simulink library "tqd"  (R2021b)
settings: Solver=VariableStepAuto  StartTime=0.0  StopTime=10.0  RelTol=1e-3
undefined symbols (not defined in the file): ATQD_AfterTqMinGain_X_Deg, ATQD_APSCreepBaseTqD_X_kph, ATQD_APSCreepBaseTqD_Y_Deg, ATQD_APSCreepBaseTqR_X_kph, ATQD_APSCreepBaseTqR_Y_Deg, ATQD_APSCreepIterm_X_kph, ATQD_APSCreepIterm_Y_kph, ATQD_APSCreepPterm_X_kph, ATQD_APSCreepPterm_Y_kph, ATQD_APSDecReq_X_kph, ATQD_APSDecReq_Y_mps2, ATQD_APSDecReqCMD_X_kph, ATQD_APSDecReqTs_X_pct, ATQD_APSDecTimeGain_X_Deg, ATQD_APSDecTimeGain_Y_s, ATQD_APSReqLowSpd_X_Deg, ATQD_AutoHoldReleaseBPS_X_Deg, ATQD_AWDLoadTrqnsGain_X_kg, ATQD_AWDLoadTrqnsGain_Y_pct, ATQD_BOSEnBPSPosn_X_kph, ATQD_BOSMap_X_rpm, ATQD_BOSMap_Y_pct, ATQD_CreepBaseTqD_X_kph, ATQD_CreepBaseTqD_Y_Deg, ATQD_CreepBaseTqR_X_kph, ATQD_CreepBaseTqR_Y_Deg, ATQD_CreepBPSDisPosn_X_Deg, ATQD_CreepBPSDisPosnR_X_Deg, ATQD_CreepBPSEnPosn_X_Deg, ATQD_CreepBPSEnPosnR_X_Deg, ATQD_CreepDeltaTq_X_kph, ATQD_CreepIterm_X_kph, ATQD_CreepIterm_Y_kph, ATQD_CreepItermMaxLimit_X_pct, ATQD_CreepPreloadTime_X_kph, ATQD_CreepPreloadTq_X_kph, ATQD_CreepPreloadTq_Y_s, ATQD_CreepProtTq_X_Deg, ATQD_CreepPterm_X_kph, ATQD_CreepPterm_Y_kph, ATQD_CreepRrTqSpRat_X_rpm, ATQD_CreepRrTqSpRat_Y_Nm, ATQD_CreepTargetSpdD_X_pct, ATQD_CreepTargetSpdR_X_pct, ATQD_ECOTqMapD_X_rpm, ATQD_ECOTqMapD_Y_pct, ATQD_EMTqMapD_X_rpm, ATQD_EMTqMapD_Y_pct, ATQD_EOPDTqMapDCon_X_rpm, ATQD_EOPDTqMapDCon_Y_Deg, ATQD_EscapeModePedTq_X_pct, ATQD_EscapeModePedTq_Y_rpm, ATQD_EscapeModePedTqFr_X_pct, ATQD_EscapeModePedTqFr_Y_rpm, ATQD_EstInitVehWeight_X_c, ATQD_FAfterTqCMDGain_X_rpm, ATQD_FAfterTqCMDGain_Y_pct, ATQD_FrLossMAPLowV_X_rpm, ATQD_FrLossMAPLowV_Y_Nm, ATQD_FrMotActReduce_X_rpm ... (+772)
libraries: simulink x211, hcu_lib x179, tqr x3
(part 16 of 28)

== system tqd/TQD/TorqueDemand/TorqueModule/OPD Hold/Deceleration Calculation ==
  VTQD_VehActSpd_kph : Inport
  VVMC_LongAcc_Gps : Inport  Port=2
  VTQD_APSReqTimer_s : Inport  Port=3
  VVMC_EstSlope_Deg : Inport  Port=4
  VTQD_APSDecReqA_flg : Inport  Port=5
  VTQD_AutiHoldRelease_flg : Inport  Port=6
  task_time_s : Inport  Port=7
  VTQD_ActAPSPosn_pct : Inport  Port=8
  AND1 : Logic  Inputs=3  AllPortsSameDT=off  OutDataTypeStr=boolean
  AND4 : Logic  Inputs=3  AllPortsSameDT=off  OutDataTypeStr=boolean
  Add : Sum  Inputs=+-
  Constant1 : Constant  Value=KTQD_APSDecReqMaxTime_s
  Constant13 : Constant  Value=ZERO_FLOAT
  Constant19 : Constant  Value=KTQD_OPDHoldBrkSW_flg
  Constant2 : Constant  Value=KTQD_OPDHoldBrkSW_flg
  Constant21 : Constant  Value=KTQD_OPDHoldDevUpLim_mps2
  Constant22 : Constant  Value=KTQD_OPDHoldDevLowLim_mps2
  Constant43 : Constant  Value=KTQD_APSDecReqMaxSW_flg
  Constant8 : Constant  Value=KVMC_GravityValue_mps2
  Delay : Delay  DelayLength=1
  FirstOrderFilter1 : tqr/TQR/Determine Torque Request/TorqueArbitrament/TorqueSmooth/FirstOrderFilter
  MTQD_APSDecReg_Z_mps2 : Lookup_n-D  BreakpointsForDimension1=ATQD_APSDecReq_Y_mps2  BreakpointsForDimension2=ATQD_APSDecReq_X_kph  Table=MTQD_APSDecReq_Z_mps2  InternalRulePriority=Speed  RndMeth=Simplest  InputSameDT=on
      settings: InputPortMap=u0,u1
  MTQD_APSDecReqCMD_Y_mps2 : Lookup_n-D  NumberOfTableDimensions=1  BreakpointsForDimension1=ATQD_APSDecReqCMD_X_kph  Table=MTQD_APSDecReqCMD_Y_mps2  InternalRulePriority=Speed  RndMeth=Simplest  InputSameDT=on
  MTQD_APSDecReqTs_Y_c : Lookup_n-D  NumberOfTableDimensions=1  BreakpointsForDimension1=ATQD_APSDecReqTs_X_pct  Table=MTQD_APSDecReqTs_Y_c  InternalRulePriority=Speed  RndMeth=Simplest  InputSameDT=on
  MTQD_APSDecTimeGain_Z_c : Lookup_n-D  BreakpointsForDimension1=ATQD_APSDecTimeGain_Y_s  BreakpointsForDimension2=ATQD_APSDecTimeGain_X_Deg  Table=MTQD_APSDecTimeGain_Z_c  InternalRulePriority=Speed  RndMeth=Simplest  InputSameDT=on
      settings: InputPortMap=u0,u1
  Max : MinMax  Function=max  Inputs=2
  NOT{1..3,5} (4 alike) : Logic  Operator=NOT  AllPortsSameDT=off  OutDataTypeStr=boolean
  OR : Logic  Operator=OR  AllPortsSameDT=off  OutDataTypeStr=boolean
  Product : Product
  Product1 : Product
  Product2 : Product
  Relational Operator : RelationalOperator  OutDataTypeStr=boolean  RndMeth=Simplest
  SR_Latch : hcu_lib/Basic_Blocks/SR_Latch
  Saturation Dynamic : simulink/Discontinuities/Saturation Dynamic  OutMin=[]  OutMax=[]  OutDataTypeStr=Inherit: Same as second input  OutDataType=fixdt(1, 16)  OutScaling=2^-10  DoSatur=off
  Switch1 : Switch  Criteria=u2 > Threshold
  Switch3 : Switch  Criteria=u2 > Threshold
  Switch9 : Switch  Criteria=u2 > Threshold
  VTQD_APSDecReq_mps2 : Outport
  wires:
  Saturation Dynamic/1 -> MTQD_APSDecReg_Z_mps2/1  "VTQD_ActOPDHoldAccDev_mps2"
  [VVMC_EstSlope_Deg] -> MTQD_APSDecTimeGain_Z_c/2
  [VTQD_APSDecTimeGain_c] -> Product2/2
  Constant21/1 -> Saturation Dynamic/1
  Product/1 -> Max/1
  Max/1 -> Switch9/1
  MTQD_APSDecReg_Z_mps2/1 -> [VTQD_MapAPSDecReg_mps2]  "VTQD_MapAPSDecReq_mps2"
  Constant13/1 -> Switch3/3
  MTQD_APSDecReqCMD_Y_mps2/1 -> [VTQD_APSDecReqCMD_mps2]  "VTQD_APSDecReqCMD_mps2"
  [VVMC_LongAcc_Gps] -> Product1/1
  [VTQD_MapAPSDecReg_mps2] -> Product2/1
  Delay/1 -> Max/2
  Constant19/1 -> NOT5/1
  Add/1 -> Saturation Dynamic/2
  [VTQD_VehActSpd_kph] -> MTQD_APSDecReg_Z_mps2/2
  [VTQD_APSReqTimer_s] -> MTQD_APSDecTimeGain_Z_c/1
  [VTQD_MapAPSDecReg_mps2] -> Product/1
  Product2/1 -> Switch9/3
  [VTQD_APSDecReq_mps2] -> Delay/1
  Product1/1 -> Add/2
  [VTQD_VehActSpd_kph] -> MTQD_APSDecReqCMD_Y_mps2/1
  MTQD_APSDecTimeGain_Z_c/1 -> [VTQD_APSDecTimeGain_c]  "VTQD_APSDecTimeGain_c"
  [VTQD_APSDecReqA_flg] -> AND4/1
  NOT5/1 -> AND4/2
  [VTQD_APSDecTimeGain_c] -> Product/2
  [VTQD_APSDecReqCMD_mps2] -> Add/1
  Constant22/1 -> Saturation Dynamic/3
  Constant8/1 -> Product1/2
  VTQD_VehActSpd_kph/1 -> [VTQD_VehActSpd_kph]
  VVMC_LongAcc_Gps/1 -> [VVMC_LongAcc_Gps]
  VTQD_APSReqTimer_s/1 -> [VTQD_APSReqTimer_s]
  VVMC_EstSlope_Deg/1 -> [VVMC_EstSlope_Deg]
  VTQD_APSDecReqA_flg/1 -> [VTQD_APSDecReqA_flg]
  [VTQD_APSDecReq_mps2] -> VTQD_APSDecReq_mps2/1
  Constant43/1 -> OR/1
  Relational Operator/1 -> SR_Latch/1
  Constant1/1 -> Relational Operator/2
  [VTQD_APSReqTimer_s] -> Relational Operator/1
  Switch9/1 -> Switch3/1
  [VTQD_AutiHoldRelease_flg] -> SR_Latch/2
  VTQD_AutiHoldRelease_flg/1 -> [VTQD_AutiHoldRelease_flg]
  OR/1 -> Switch9/2  "VTQD_APSDecReqMax_flg"
  SR_Latch/1 -> OR/2
  AND4/1 -> Switch3/2
  NOT2/1 -> AND4/3
  [VTQD_AutiHoldRelease_flg] -> NOT2/1
  NOT1/1 -> AND1/3
  NOT3/1 -> AND1/2
  AND1/1 -> Switch1/2
  Switch3/1 -> Switch1/1, FirstOrderFilter1/1
  Switch1/1 -> [VTQD_APSDecReq_mps2]  "VTQD_APSDecReq_mps2"
  [VTQD_APSDecReqA_flg] -> AND1/1
  Constant2/1 -> NOT3/1
  [VTQD_AutiHoldRelease_flg] -> NOT1/1
  FirstOrderFilter1/1 -> Switch1/3
  [task_time_s] -> FirstOrderFilter1/2
  task_time_s/1 -> [task_time_s]
  VTQD_ActAPSPosn_pct/1 -> [VTQD_ActAPSPosn_pct]
  MTQD_APSDecReqTs_Y_c/1 -> [VTQD_APSDecReqTs_c]  "VTQD_APSDecReqTs_c"
  [VTQD_ActAPSPosn_pct] -> MTQD_APSDecReqTs_Y_c/1
  [VTQD_APSDecReqTs_c] -> FirstOrderFilter1/3

== system tqd/TQD/TorqueDemand/TorqueModule/OPD Hold/OPDHold Request  ==
  VTQD_VehActSpd_kph : Inport
  VTQD_APSStaSys_enum : Inport  Port=2
  VTQD_AutiHoldRelease_flg : Inport  Port=3
  task_time_s : Inport  Port=4
  VVMC_EstSlope_Deg : Inport  Port=5
  AND : Logic  AllPortsSameDT=off  OutDataTypeStr=boolean
  AND1 : Logic  Inputs=3  AllPortsSameDT=off  OutDataTypeStr=boolean
  AND2 : Logic  Operator=OR  AllPortsSameDT=off  OutDataTypeStr=boolean
  AND3 : Logic  AllPortsSameDT=off  OutDataTypeStr=boolean
  Constant1 : Constant  Value=KTQD_APSReqUpSpd_kph
  Constant10 : Constant  Value=KTQD_APSReqDownSpd_kph
  Constant11 : Constant  Value=KTQD_OPDHoldLampDelayTime_s
  Constant12 : Constant  Value=KTQD_OPDHoldLampEnSpd_kph  OutDataTypeStr=single
  Constant13 : Constant  Value=KTQD_OPDHoldLampDisSpd_kph  OutDataTypeStr=single
  Constant2 : Constant  Value=2  OutDataTypeStr=uint8
  Constant3 : Constant  Value=2  OutDataTypeStr=uint8
  Constant4 : Constant  OutDataTypeStr=uint8
  Constant5 : Constant  Value=2  OutDataTypeStr=uint8
  Constant6 : Constant  Value=0  OutDataTypeStr=uint8
  Constant7 : Constant  OutDataTypeStr=uint8
  Constant8 : Constant  OutDataTypeStr=uint8
  Constant9 : Constant  Value=KTQD_APSReqDelayTime_s
  Equal1 : RelationalOperator  Operator=<  OutDataTypeStr=boolean  RndMeth=Simplest
  Equal2 : RelationalOperator  Operator=~=  OutDataTypeStr=boolean  RndMeth=Simplest
  Equal3 : RelationalOperator  Operator===  OutDataTypeStr=boolean  RndMeth=Simplest
  Equal4 : RelationalOperator  Operator===  OutDataTypeStr=boolean  RndMeth=Simplest
  Equal5 : RelationalOperator  Operator===  OutDataTypeStr=boolean  RndMeth=Simplest
  Equal6 : RelationalOperator  Operator=>  OutDataTypeStr=boolean  RndMeth=Simplest
  MTQD_APSReqLowSpd_Y_kph : Lookup_n-D  NumberOfTableDimensions=1  BreakpointsForDimension1=ATQD_APSReqLowSpd_X_Deg  Table=MTQD_APSReqLowSpd_Y_kph  InternalRulePriority=Speed  RndMeth=Simplest  InputSameDT=on
  NOT1 : Logic  Operator=NOT  AllPortsSameDT=off  OutDataTypeStr=boolean
  NOT2 : Logic  Operator=NOT  AllPortsSameDT=off  OutDataTypeStr=boolean
  Relational Operator1 : RelationalOperator  Operator=<  OutDataTypeStr=boolean  RndMeth=Simplest
  Relational Operator2 : RelationalOperator  OutDataTypeStr=boolean  RndMeth=Simplest
  Relational Operator3 : RelationalOperator  Operator=<  OutDataTypeStr=boolean  RndMeth=Simplest
  Relational Operator4 : RelationalOperator  Operator=>  OutDataTypeStr=boolean  RndMeth=Simplest
  Relay : Relay  OnSwitchValue=KTQD_OPDHoldGradeUp_Deg  OffSwitchValue=KTQD_OPDHoldGradeDown_Deg  OutDataTypeStr=boolean
  SR_Latch : hcu_lib/Basic_Blocks/SR_Latch
  SR_Latch1 : hcu_lib/Basic_Blocks/SR_Latch
  Switch : Switch  Criteria=u2 > Threshold
  Switch1 : Switch  Criteria=u2 > Threshold
  Switch2 : Switch  Criteria=u2 > Threshold
  Timer : hcu_lib/Basic_Blocks/Timer
  VTQD_APSReqTimer_s : Outport
  VTQD_APSReq_enum : Outport  Port=2
  VTQD_APSDecReqA_flg : Outport  Port=3
  VTQD_OPDHoldLamp_flg : Outport  Port=4
  wires:
  [task_time_s] -> Timer/3
  Constant4/1 -> Switch1/1
  NOT2/1 -> Timer/2
  Switch2/1 -> [VTQD_APSReq_enum]  "VTQD_APSReq_enum"
  AND/1 -> Switch1/2  "VTQD_APSStasysUp_flg"
  Constant9/1 -> Relational Operator2/2, Timer/4
  Equal3/1 -> AND/2
  Constant6/1 -> Switch1/3
  Timer/1 -> [VTQD_APSReqTimer_s], Relational Operator2/1  "VTQD_APSReqTimer_s"
  Relational Operator2/1 -> Switch2/2
  Constant8/1 -> Switch2/1
  Equal4/1 -> AND1/2
  [VTQD_APSStaSys_enum] -> Equal3/1
  [VTQD_VehActSpd_kph] -> Equal1/1
  Equal5/1 -> [VTQD_APSDecReqA_flg]  "VTQD_APSDecReqA_flg"
  [VTQD_APSReqUpSpd_kph] -> Equal1/2
  NOT1/1 -> AND1/3
  Constant7/1 -> Equal5/2
  [VTQD_APSReq_enum] -> Equal5/1
  Constant2/1 -> Equal3/2
  Switch1/1 -> Switch2/3
  Equal1/1 -> AND/1
  [VTQD_APSStaSys_enum] -> Equal4/1
  [VTQD_VehActSpd_kph] -> Relational Operator1/1
  AND1/1 -> NOT2/1, Timer/1  "VTQD_APSStasysLow_flg"
  Constant5/1 -> Equal4/2
  VTQD_VehActSpd_kph/1 -> [VTQD_VehActSpd_kph]
  VTQD_APSStaSys_enum/1 -> [VTQD_APSStaSys_enum]
  VTQD_AutiHoldRelease_flg/1 -> [VTQD_AutiHoldRelease_flg]
  task_time_s/1 -> [task_time_s]
  [VTQD_APSReqTimer_s] -> VTQD_APSReqTimer_s/1
  [VTQD_APSReq_enum] -> VTQD_APSReq_enum/1
  [VTQD_APSDecReqA_flg] -> VTQD_APSDecReqA_flg/1
  [VTQD_AutiHoldRelease_flg] -> NOT1/1
  VVMC_EstSlope_Deg/1 -> [VVMC_EstSlope_Deg]
  MTQD_APSReqLowSpd_Y_kph/1 -> Relational Operator1/2  "VTQD_APSReqLowSpd_kph"
  [VVMC_EstSlope_Deg] -> MTQD_APSReqLowSpd_Y_kph/1
  SR_Latch/1 -> AND1/1
  Relational Operator1/1 -> SR_Latch/1
  AND2/1 -> SR_Latch/2
  [VTQD_AutiHoldRelease_flg] -> AND2/1
  Constant3/1 -> Equal2/2
  [VTQD_APSStaSys_enum] -> Equal2/1
  Equal2/1 -> AND2/2
  [VVMC_EstSlope_Deg] -> Relay/1
  Relay/1 -> Switch/2  "VTQD_OPDHoldUpDown_flg"
  Constant1/1 -> Switch/1
  Constant10/1 -> Switch/3
  Switch/1 -> [VTQD_APSReqUpSpd_kph]  "VTQD_APSReqUpSpd_kph"
  Constant11/1 -> Equal6/2
  [VTQD_APSReqTimer_s] -> Equal6/1
  [VTQD_OPDHoldLamp_flg] -> VTQD_OPDHoldLamp_flg/1
  [VTQD_VehActSpd_kph] -> Relational Operator3/1
  Relational Operator3/1 -> SR_Latch1/1
  Constant12/1 -> Relational Operator3/2
  [VTQD_VehActSpd_kph] -> Relational Operator4/1
  Constant13/1 -> Relational Operator4/2
  Relational Operator4/1 -> SR_Latch1/2
  Equal6/1 -> AND3/1
  SR_Latch1/1 -> AND3/2  "VTQD_OPDHoldSpdEnLamp_flg"
  AND3/1 -> [VTQD_OPDHoldLamp_flg]  "VTQD_OPDHoldLamp_flg"

== system tqd/TQD/TorqueDemand/TorqueModule/OPD Hold/Parking Requeest Backup ==
  VTQD_APSReq_enum : Inport
  VTQD_APSReqTimer_s : Inport  Port=2
  VTQD_ParkRequest_flg : Inport  Port=3
  task_time_s : Inport  Port=4
  VTQD_AutiHoldRelease_flg : Inport  Port=5
  AND : Logic  AllPortsSameDT=off  OutDataTypeStr=boolean
  AND1 : Logic  AllPortsSameDT=off  OutDataTypeStr=boolean
  AND3 : Logic  Inputs=3  AllPortsSameDT=off  OutDataTypeStr=boolean
  Constant1 : Constant  Value=KTQD_APSReqDelayTime_s
  Constant16 : Constant  OutDataTypeStr=uint8
  Constant17 : Constant  Value=TRUE  OutDataTypeStr=uint8
  Constant2 : Constant  Value=KTQD_APSReqDelayTime_s
  Constant3 : Constant  Value=KTQD_OPDHoldBrkSW_flg
  Constant4 : Constant  Value=KTQD_OPDHoldAllowPark_flg
  Constant5 : Constant  Value=KTQD_OPDHoldAllowPark_s
  Constant6 : Constant  Value=KTQD_OPDHoldAllowGearPSW_flg
  DelayEnable : hcu_lib/Basic_Blocks/DelayEnable
  Equal6 : RelationalOperator  Operator===  OutDataTypeStr=boolean  RndMeth=Simplest
  NOT : Logic  Operator=NOT  AllPortsSameDT=off  OutDataTypeStr=boolean
  OR : Logic  Operator=OR  AllPortsSameDT=off  OutDataTypeStr=boolean
  Relational Operator1 : RelationalOperator  OutDataTypeStr=boolean  RndMeth=Simplest
  Relational Operator6 : RelationalOperator  OutDataTypeStr=boolean  RndMeth=Simplest
  SR_Latch : hcu_lib/Basic_Blocks/SR_Latch
  Switch4 : Switch  Criteria=u2 > Threshold
  VTQD_ActParkRequest_flg : Outport
  VTQD_OPDHoldAllowPark_flg : Outport  Port=2
  wires:
  Constant3/1 -> AND3/2
  Constant1/1 -> Relational Operator6/2
  Equal6/1 -> AND3/1
  [VTQD_APSReq_enum] -> Equal6/1
  Relational Operator6/1 -> AND3/3
  [VTQD_ParkRequest_flg] -> Switch4/3
  Constant17/1 -> Switch4/1
  Constant16/1 -> Equal6/2
  Switch4/1 -> [VTQD_ActParkRequest_flg]  "VTQD_ActParkRequest_flg"
  [VTQD_APSReqTimer_s] -> Relational Operator6/1
  VTQD_APSReq_enum/1 -> [VTQD_APSReq_enum]
  VTQD_APSReqTimer_s/1 -> [VTQD_APSReqTimer_s]
  VTQD_ParkRequest_flg/1 -> [VTQD_ParkRequest_flg]
  [VTQD_ActParkRequest_flg] -> VTQD_ActParkRequest_flg/1
  Constant2/1 -> Relational Operator1/2
  [VTQD_APSReqTimer_s] -> Relational Operator1/1
  task_time_s/1 -> [task_time_s]
  AND/1 -> DelayEnable/1
  Relational Operator1/1 -> AND/1
  Constant4/1 -> AND/2
  Constant5/1 -> DelayEnable/2
  DelayEnable/1 -> SR_Latch/1
  [VTQD_AutiHoldRelease_flg] -> SR_Latch/2
  VTQD_AutiHoldRelease_flg/1 -> [VTQD_AutiHoldRelease_flg]
  SR_Latch/1 -> [VTQD_OPDHoldAllowPark_flg]  "VTQD_OPDHoldAllowPark_flg"
  OR/1 -> Switch4/2
  AND3/1 -> OR/1
  [task_time_s] -> DelayEnable/3
  [VTQD_OPDHoldAllowPark_flg] -> AND1/1
  AND1/1 -> OR/2
  NOT/1 -> AND1/2
  Constant6/1 -> NOT/1
  [VTQD_OPDHoldAllowPark_flg] -> VTQD_OPDHoldAllowPark_flg/1

== system tqd/TQD/TorqueDemand/TorqueModule/OPD Hold/Release Condition ==
  VVMC_EstSlope_Deg : Inport
  VTQD_VehActSpd_kph : Inport  Port=2
  VTQR_NoABSFEDUWhlTqReq_Nm : Inport  Port=3
  VTQR_NoABSREDUWhlTqReq_Nm : Inport  Port=4
  VTQD_ActBPSPosn_pct : Inport  Port=5
  task_time_s : Inport  Port=6
  VTQD_APSReqTimer_s : Inport  Port=7
  VTQD_LowIdleAccPedal_flg : Inport  Port=8
  VTQD_OPDHoldRgnOn2Off_flg : Inport  Port=9
  AND : Logic  Inputs=3  AllPortsSameDT=off  OutDataTypeStr=boolean
  AND1 : Logic  AllPortsSameDT=off  OutDataTypeStr=boolean
  AND2 : Logic  AllPortsSameDT=off  OutDataTypeStr=boolean
  AND3 : Logic  AllPortsSameDT=off  OutDataTypeStr=boolean
  Add : Sum
  Add1 : Sum  Inputs=+-+
  Add6 : Sum
  Add7 : Sum
  Constant1 : Constant  Value=KTQD_APSRelDisTqDev_Nm
  Constant{5,10,23,30} (4 alike) : Constant  Value=ZERO_FLOAT
  Constant2 : Constant  Value=KTQD_OPDHoldDownEnTime_s
  Constant36 : Constant  Value=KTQD_OPDHoldRelDetSpd_kph
  Constant4 : Constant  Value=KTQD_OPDHoldRelTqGain_Nm
  Constant6 : Constant  Value=KTQD_OPDHoldDetRevSpd_kph
  Constant7 : Constant  Value=KTQD_OPDHoldLiftRevSpd_kph
  Constant8 : Constant  Value=KTQD_APSDecReqMaxTime_s
  Constant9 : Constant  Value=KTQD_OPDHoldRelTqGain_Nm
  Delay{,1..3} (4 alike) : Delay  DelayLength=1
  DelayEnable : hcu_lib/Basic_Blocks/DelayEnable
  DelayEnable1 : hcu_lib/Basic_Blocks/DelayEnable
  Detect Increase : simulink/Logic and Bit Operations/Detect Increase  vinit=0.0  OutDataTypeStr=boolean
  Detect Increase1 : simulink/Logic and Bit Operations/Detect Increase  vinit=0.0  OutDataTypeStr=boolean
  Detect Increase2 : simulink/Logic and Bit Operations/Detect Increase  vinit=0.0  OutDataTypeStr=boolean
  MTQD_AutoHoldReleaseBPS_Y_pct : Lookup_n-D  NumberOfTableDimensions=1  BreakpointsForDimension1=ATQD_AutoHoldReleaseBPS_X_Deg  Table=MTQD_AutoHoldReleaseBPS_Y_pct  InternalRulePriority=Speed  RndMeth=Simplest  InputSameDT=on
  MTQD_OPDHoldDownRelDelay_Y_s : Lookup_n-D  NumberOfTableDimensions=1  BreakpointsForDimension1=ATQD_OPDHoldDownRelDelay_X_Deg  Table=MTQD_OPDHoldDownRelDelay_Y_s  InternalRulePriority=Speed  RndMeth=Simplest  InputSameDT=on
  MTQD_OPDHoldRelDetTime_Y_s : Lookup_n-D  NumberOfTableDimensions=1  BreakpointsForDimension1=ATQD_OPDHoldRelDetTime_X_Deg  Table=MTQD_OPDHoldRelDetTime_Y_s  InternalRulePriority=Speed  RndMeth=Simplest  InputSameDT=on
  MTQD_OPDHoldReleaseTq_Y_Nm{,1..3} (4 alike) : Lookup_n-D  NumberOfTableDimensions=1  BreakpointsForDimension1=ATQD_OPDHoldReleaseTq_X_Deg  Table=MTQD_OPDHoldReleaseTq_Y_Nm  InternalRulePriority=Speed  RndMeth=Simplest  InputSameDT=on
  Max : MinMax  Function=max  Inputs=2
  Max1 : MinMax  Function=max  Inputs=2
  Max2 : MinMax  Function=max  Inputs=2
  NOT{,1..5} (6 alike) : Logic  Operator=NOT  AllPortsSameDT=off  OutDataTypeStr=boolean
  OR : Logic  Operator=OR  AllPortsSameDT=off  OutDataTypeStr=boolean
  OR1 : Logic  Operator=OR  AllPortsSameDT=off  OutDataTypeStr=boolean
  OR2 : Logic  Operator=OR  AllPortsSameDT=off  OutDataTypeStr=boolean
  OR3 : Logic  Operator=OR  Inputs=3  AllPortsSameDT=off  OutDataTypeStr=boolean
  Relational Operator : RelationalOperator  Operator=>  OutDataTypeStr=boolean  RndMeth=Simplest
  Relational Operator1 : RelationalOperator  Operator=<=  OutDataTypeStr=boolean  RndMeth=Simplest
  Relational Operator3 : RelationalOperator  Operator=<=  OutDataTypeStr=boolean  RndMeth=Simplest
  Relational Operator4 : RelationalOperator  OutDataTypeStr=boolean  RndMeth=Simplest
  Relational Operator5 : RelationalOperator  Operator=<  OutDataTypeStr=boolean  RndMeth=Simplest
  Relational Operator6 : RelationalOperator  Operator=>  OutDataTypeStr=boolean  RndMeth=Simplest
  Relational Operator7 : RelationalOperator  OutDataTypeStr=boolean  RndMeth=Simplest
  Relational Operator9 : RelationalOperator  OutDataTypeStr=boolean  RndMeth=Simplest
  Relay : Relay  OnSwitchValue=KTQD_OPDHoldGradeUp_Deg  OffSwitchValue=KTQD_OPDHoldGradeDown_Deg  OutDataTypeStr=boolean
  Relay1 : Relay  OnSwitchValue=KTQD_OPDHoldGradeUp_Deg  OffSwitchValue=KTQD_OPDHoldGradeDown_Deg  OutDataTypeStr=boolean
  SR_Latch : hcu_lib/Basic_Blocks/SR_Latch
  SR_Latch1 : hcu_lib/Basic_Blocks/SR_Latch
  Switch{,1..6} (7 alike) : Switch  Criteria=u2 > Threshold
  VTQD_AutoHoldRelease_flg : Outport
  VTQD_OPDHoldEnRel_flg : Outport  Port=2
  VTQD_OPDHoldActRelTq_Nm : Outport  Port=3
  wires:
  VVMC_EstSlope_Deg/1 -> [VVMC_EstSlope_Deg]
  VTQD_VehActSpd_kph/1 -> [VTQD_VehActSpd_kph]
  VTQR_NoABSFEDUWhlTqReq_Nm/1 -> [VTQR_NoABSFEDUWhlTqReq_Nm]
  VTQR_NoABSREDUWhlTqReq_Nm/1 -> [VTQR_NoABSREDUWhlTqReq_Nm]
  VTQD_ActBPSPosn_pct/1 -> [VTQD_ActBPSPosn_pct]
  task_time_s/1 -> [task_time_s]
  [VTQD_AutoHoldRelease_flg] -> VTQD_AutoHoldRelease_flg/1
  [VTQD_OPDHoldEnRel_flg] -> VTQD_OPDHoldEnRel_flg/1
  VTQD_APSReqTimer_s/1 -> [VTQD_APSReqTimer_s]
  VTQD_LowIdleAccPedal_flg/1 -> [VTQD_LowIdleAccPedal_flg]
  VTQD_OPDHoldRgnOn2Off_flg/1 -> [VTQD_OPDHoldRgnOn2Off_flg]
  SR_Latch/1 -> DelayEnable/1  "VTQD_OPDHoldEnRelLatch_flg"
  Detect Increase2/1 -> OR2/1
  Detect Increase1/1 -> SR_Latch1/1
  DelayEnable1/1 -> Switch1/1
  SR_Latch1/1 -> [VTQD_OPDHoldRelReverse_flg]  "VTQD_OPDHoldRelReverse_flg"
  MTQD_OPDHoldDownRelDelay_Y_s/1 -> [VTQD_OPDHoldDownRelDelay_s]  "VTQD_OPDHoldDownRelDelay_s"
  Constant4/1 -> Switch2/1
  [VVMC_EstSlope_Deg] -> MTQD_OPDHoldDownRelDelay_Y_s/1
  [task_time_s] -> DelayEnable1/3
  [VTQD_LowIdleAccPedal_flg] -> NOT2/1
  Constant30/1 -> Switch5/1
  NOT/1 -> AND/2
  [VVMC_EstSlope_Deg] -> Relay1/1
  Relay1/1 -> NOT3/1
  Constant2/1 -> Relational Operator1/2
  OR1/1 -> AND/3
  Switch1/1 -> Switch/3
  AND2/1 -> Switch1/3
  [VTQD_LowIdleAccPedal_flg] -> NOT1/1
  [VTQD_OPDHoldRgnOn2Off_flg] -> Switch/2
  Relational Operator/1 -> OR1/1
  Relational Operator1/1 -> AND/1
  [VTQD_OPDHoldRelDetTime_s] -> DelayEnable/2
  AND/1 -> OR/1
  [VVMC_EstSlope_Deg] -> Relay/1
  [VTQR_NoABSFEDUWhlTqReq_Nm] -> Add6/1
  [VTQR_NoABSREDUWhlTqReq_Nm] -> Add6/2
  [task_time_s] -> DelayEnable/3
  [VTQR_NoABSFEDUWhlTqReq_Nm] -> Add7/1
  [VTQD_ActBPSPosn_pct] -> Relational Operator/1
  Add1/1 -> Max1/1
  [VVMC_EstSlope_Deg] -> MTQD_OPDHoldReleaseTq_Y_Nm/1
  DelayEnable/1 -> [VTQD_OPDHoldEnRel_flg]  "VTQD_OPDHoldEnRel_flg"
  [VTQR_NoABSREDUWhlTqReq_Nm] -> Add7/2
  Max1/1 -> Relational Operator5/2
  [VTQD_VehActSpd_kph] -> Relational Operator9/1
  Relational Operator9/1 -> Switch5/2
  [VVMC_EstSlope_Deg] -> MTQD_AutoHoldReleaseBPS_Y_pct/1
  [VVMC_EstSlope_Deg] -> MTQD_OPDHoldRelDetTime_Y_s/1
  Switch5/1 -> [VTQD_OPDHoldRelDetTime_s]  "VTQD_OPDHoldRelDetTime_s"
  MTQD_AutoHoldReleaseBPS_Y_pct/1 -> Relational Operator/2  "VTQD_AutoHoldReleaseAPS_pct"
  OR/1 -> [VTQD_AutoHoldRelease_flg]  "VTQD_AutoHoldRelease_flg"
  MTQD_OPDHoldReleaseTq_Y_Nm/1 -> Switch6/3
  Relational Operator3/1 -> Detect Increase1/1
  [VTQD_OPDHoldDownRelDelay_s] -> DelayEnable1/2
  Delay3/1 -> Max2/1
  Max2/1 -> Switch6/1
  Constant6/1 -> Relational Operator3/2
  Detect Increase/1 -> OR3/1
  Add7/1 -> Relational Operator5/1  "VTQD_OPDHoldDisRelTq_Nm"
  Switch6/1 -> Add/2, Delay3/1  "VTQD_OPDHoldReleaseTq_Nm"
  [VVMC_EstSlope_Deg] -> MTQD_OPDHoldReleaseTq_Y_Nm3/1
  [VTQD_APSReqTimer_s] -> Delay/1
  NOT3/1 -> Switch1/2
  [VTQD_OPDHoldRelReverse_flg] -> Detect Increase2/1
  [VTQD_OPDHoldRelReverse_flg] -> Switch6/2
  Constant23/1 -> Max1/2
  [VTQD_LowIdleAccPedal_flg] -> NOT4/1
  MTQD_OPDHoldRelDetTime_Y_s/1 -> Switch5/3
  [VTQD_OPDHoldRelReverse_flg] -> Switch3/2
  Relational Operator4/1 -> SR_Latch/1  "VTQD_OPDHoldEnRelease_flg"
  Switch2/1 -> Add/1
  NOT5/1 -> AND2/2
  MTQD_OPDHoldReleaseTq_Y_Nm1/1 -> Switch4/3
  Relay/1 -> NOT/1
  Add/1 -> [VTQD_OPDHoldActRelTq_Nm], Relational Operator4/2  "VTQD_OPDHoldActRelTq_Nm"
  [VTQD_OPDHoldRelReverse_flg] -> Switch4/2
  Delay/1 -> Relational Operator1/1
  Constant8/1 -> Relational Operator7/2
  OR2/1 -> SR_Latch/2
  [VTQD_VehActSpd_kph] -> Relational Operator3/1
  Delay2/1 -> Max/1
  [VTQD_OPDHoldEnRel_flg] -> AND1/2
  AND1/1 -> Switch/1
  [VTQD_LowIdleAccPedal_flg] -> AND3/1
  [VTQD_LowIdleAccPedal_flg] -> NOT5/1
  Constant36/1 -> Relational Operator9/2
  NOT4/1 -> DelayEnable1/1
  [VTQD_APSReqTimer_s] -> Delay1/1
  Constant10/1 -> Switch3/3
  MTQD_OPDHoldReleaseTq_Y_Nm2/1 -> Max/2
  [VTQD_LowIdleAccPedal_flg] -> Detect Increase/1
  Add6/1 -> Relational Operator4/1  "VTQD_OPDHoldEnRelTq_Nm"
  [VTQD_OPDHoldRelReverse_flg] -> Switch2/2
  Switch3/1 -> Add1/1
  [VVMC_EstSlope_Deg] -> MTQD_OPDHoldReleaseTq_Y_Nm1/1
  Relational Operator5/1 -> OR2/2  "VTQD_OPDHoldDisRelease_flg"
  MTQD_OPDHoldReleaseTq_Y_Nm3/1 -> Max2/2
  Delay1/1 -> Relational Operator7/1
  Relational Operator7/1 -> AND3/2
  Constant7/1 -> Relational Operator6/2
  Switch4/1 -> Delay2/1, Add1/3
  Constant5/1 -> Switch2/3
  AND3/1 -> OR3/3
  Constant9/1 -> Switch3/1
  Switch/1 -> OR/2
  NOT2/1 -> AND1/1
  [VTQD_VehActSpd_kph] -> Relational Operator6/1
  [VTQD_OPDHoldEnRel_flg] -> AND2/1
  Constant1/1 -> Add1/2
  NOT1/1 -> OR1/2
  Relational Operator6/1 -> OR3/2
  Max/1 -> Switch4/1
  [VVMC_EstSlope_Deg] -> MTQD_OPDHoldReleaseTq_Y_Nm2/1
  OR3/1 -> SR_Latch1/2
  [VTQD_OPDHoldActRelTq_Nm] -> VTQD_OPDHoldActRelTq_Nm/1

== system tqd/TQD/TorqueDemand/TorqueModule/OPD Hold/System Status ==
  VTQD_GearActualPosn_enum : Inport
  VINP_EPBSta_enum : Inport  Port=2
  VTQD_RegenMode_enum : Inport  Port=3
  VTQD_AutiHoldRelease_flg : Inport  Port=4
  VVMC_ADASActive_flg : Inport  Port=5
  VPMM_PwrSta_enum : Inport  Port=6
  VVMC_CruzActive_flg : Inport  Port=7
  VTQD_VehActSpd_kph : Inport  Port=8
  VVMC_EstSlope_Deg : Inport  Port=9
  task_time_s : Inport  Port=10
  VINP_FrPTCSActive_flg : Inport  Port=11
  VINP_RrPTCSActive_flg : Inport  Port=12
  VINP_ESCActive_flg : Inport  Port=13
  VINP_ABSActive_flg : Inport  Port=14
  VVMC_APSActive_flg : Inport  Port=15
  VTQD_PedAccTqEn_flg : Inport  Port=16
  VINP_IVICreepOnSW_flg : Inport  Port=17
  VTQD_IVIRockModeEn_flg : Inport  Port=18
  VTQD_ActWhlSkipSta_enum : Inport  Port=19
  VTQD_SkipDirect_enum : Inport  Port=20
  VTQD_LimpHomeAct_flg : Inport  Port=21
  AND{,3..7,9} (7 alike) : Logic  AllPortsSameDT=off  OutDataTypeStr=boolean
  AND1 : Logic  Inputs=4  AllPortsSameDT=off  OutDataTypeStr=boolean
  AND2 : Logic  Inputs=14  AllPortsSameDT=off  OutDataTypeStr=boolean
  AND8 : Logic  Inputs=3  AllPortsSameDT=off  OutDataTypeStr=boolean
  Constant1 : Constant  Value=2  OutDataTypeStr=uint8
  Constant10 : Constant  Value=ENUM_GEARACTUALPOSN_R
  Constant11 : Constant  Value=ENUM_GEARACTUALPOSN_D
  Constant12 : Constant  Value=KTQD_R2DGradeUpLim_Deg
  Constant13 : Constant  Value=KTQD_R2DGradeLowLim_Deg
  Constant14 : Constant  Value=KTQD_R2DEnOPDHoldSpd_kph
  Constant15 : Constant  Value=KTQD_R2DEnOPDHSpdDelayTime_s
  Constant16 : Constant  Value=ENUM_SKIPDISOPDHOLD_HIGH
  Constant17 : Constant  Value=ENUM_SKIPDIRECT_NEGATIVE
  Constant18 : Constant  Value=KTQD_OPDHoldSkipDetSpd_kph
  Constant19 : Constant  Value=ENUM_SKIPDISOPDHOLD_NORMAL
  Constant2 : Constant  Value=0  OutDataTypeStr=uint8
  Constant20 : Constant  Value=ENUM_GEARACTUALPOSN_P
  Constant21 : Constant  Value=ENUM_GEARACTUALPOSN_N
  Constant22 : Constant  Value=KTQD_SkipRecOPDHoldDelay_s
  Constant23 : Constant  Value=KTQD_OPDHoldSkipDetSpd_kph
  Constant3 : Constant  Value=ENUM_EPBSTA_APPLIED
  Constant4 : Constant  Value=ENUM_GEARACTUALPOSN_P
  Constant40 : Constant  Value=ENUM_REGENLEVEL_OPD
  Constant44 : Constant  Value=ENUM_REGENLEVEL_OPD
  Constant45 : Constant  Value=ENUM_POWERSTA_READY
  Constant5 : Constant  Value=ENUM_GEARACTUALPOSN_D
  Constant6 : Constant  Value=KTQD_AutoHoldEnSpd_kph
  Constant7 : Constant  Value=ENUM_EPBSTA_APPLIED
  Constant8 : Constant  Value=ENUM_REGENLEVEL_OPD
  Constant9 : Constant  Value=ENUM_GEARACTUALPOSN_P
  Delay : Delay  DelayLength=1
  Delay2 : Delay  DelayLength=1
  Delay3 : Delay  DelayLength=1
  DelayEnable : hcu_lib/Basic_Blocks/DelayEnable
  DelayEnable1 : hcu_lib/Basic_Blocks/DelayEnable
  Equal{,1..2,5..9,11,13..15,30} (13 alike) : RelationalOperator  Operator===  OutDataTypeStr=boolean  RndMeth=Simplest
  Equal10 : RelationalOperator  Operator=~=  OutDataTypeStr=boolean  RndMeth=Simplest
  Equal3 : RelationalOperator  Operator=~=  OutDataTypeStr=boolean  RndMeth=Simplest
  Equal4 : RelationalOperator  Operator=~=  OutDataTypeStr=boolean  RndMeth=Simplest
  GreaterThan3 : RelationalOperator  Operator=>  OutDataTypeStr=boolean  RndMeth=Simplest
  MTQD_WhlSkipDisOPDHold_Y_enum : Lookup_n-D  NumberOfTableDimensions=1  BreakpointsForDimension1=ATQD_WhlSkipDisOPDHold_X_enum  BreakpointsForDimension1DataTypeStr=uint8  Table=MTQD_WhlSkipDisOPDHold_Y_enum  TableDataTypeStr=uint8  IntermediateResultsDataTypeStr=uint8  ExtrapMethod=Clip  UseLastTableValue=on  InternalRulePriority=Speed  OutDataTypeStr=uint8  RndMeth=Simplest  InputSameDT=on
  NOT{,1..11} (12 alike) : Logic  Operator=NOT  AllPortsSameDT=off  OutDataTypeStr=boolean
  OR : Logic  Operator=OR  AllPortsSameDT=off  OutDataTypeStr=boolean
  OR1 : Logic  Operator=OR  AllPortsSameDT=off  OutDataTypeStr=boolean
  OR3 : Logic  Operator=OR  Inputs=3  AllPortsSameDT=off  OutDataTypeStr=boolean
  OR5 : Logic  Operator=OR  Inputs=3  AllPortsSameDT=off  OutDataTypeStr=boolean
  Relational Operator : RelationalOperator  Operator=<=  OutDataTypeStr=boolean  RndMeth=Simplest
  Relational Operator1 : RelationalOperator  OutDataTypeStr=boolean  RndMeth=Simplest
  Relational Operator2 : RelationalOperator  OutDataTypeStr=boolean  RndMeth=Simplest
  Relational Operator3 : RelationalOperator  Operator=<=  OutDataTypeStr=boolean  RndMeth=Simplest
  Relational Operator4 : RelationalOperator  Operator=<=  OutDataTypeStr=boolean  RndMeth=Simplest
  Relational Operator5 : RelationalOperator  Operator=>  OutDataTypeStr=boolean  RndMeth=Simplest
  SR_Latch : hcu_lib/Basic_Blocks/SR_Latch
  SR_Latch3 : hcu_lib/Basic_Blocks/SR_Latch
  SR_Latch4 : hcu_lib/Basic_Blocks/SR_Latch
  Switch : Switch  Criteria=u2 > Threshold
  Unit Delay1 : UnitDelay  SampleTime=-1  HasFrameUpgradeWarning=on
  VTQD_APSStaSys_enum : Outport
  VTQD_OPDHoldDelayForP_flg : Outport  Port=2
  VTQD_OPDHoldRgnOn2Off_flg : Outport  Port=3
  wires:
  Switch/1 -> [VTQD_APSStaSys_enum]  "VTQD_APSStaSys_enum"
  Constant2/1 -> Switch/3
  AND2/1 -> Switch/2
  Constant1/1 -> Switch/1
  [VTQD_GearActualPosn_enum] -> Equal1/1
  Equal1/1 -> AND5/1
  AND5/1 -> [VTQD_OPDHoldDelayForP_flg]  "VTQD_OPDHoldDelayForP_flg"
  Equal10/1 -> AND5/2
  Equal11/1 -> GreaterThan3/2, Unit Delay1/1
  SR_Latch3/1 -> [VTQD_OPDHoldRgnOn2Off_flg]  "VTQD_OPDHoldRgnOn2Off_flg"
  GreaterThan3/1 -> AND6/2
  Constant45/1 -> Equal30/2
  AND6/1 -> SR_Latch3/1
  [VPMM_PwrSta_enum] -> Equal30/1
  Equal30/1 -> AND6/1
  Unit Delay1/1 -> GreaterThan3/1
  [VTQD_AutiHoldRelease_flg] -> Delay/1
  Constant44/1 -> Equal11/2
  [VTQD_RegenMode_enum] -> Equal11/1
  Constant3/1 -> Equal10/2
  [VINP_EPBSta_enum] -> Equal10/1
  Constant4/1 -> Equal1/2
  VTQD_GearActualPosn_enum/1 -> [VTQD_GearActualPosn_enum]
  VINP_EPBSta_enum/1 -> [VINP_EPBSta_enum]
  VTQD_RegenMode_enum/1 -> [VTQD_RegenMode_enum]
  VTQD_AutiHoldRelease_flg/1 -> [VTQD_AutiHoldRelease_flg]
  VVMC_ADASActive_flg/1 -> [VVMC_ADASActive_flg]
  VPMM_PwrSta_enum/1 -> [VPMM_PwrSta_enum]
  VVMC_CruzActive_flg/1 -> [VVMC_CruzActive_flg]
  VTQD_VehActSpd_kph/1 -> [VTQD_VehActSpd_kph]
  [VTQD_APSStaSys_enum] -> VTQD_APSStaSys_enum/1
  [VTQD_OPDHoldDelayForP_flg] -> VTQD_OPDHoldDelayForP_flg/1
  [VTQD_OPDHoldRgnOn2Off_flg] -> VTQD_OPDHoldRgnOn2Off_flg/1
  Constant9/1 -> Equal5/2
  Equal4/1 -> AND/1
  [VTQD_GearActualPosn_enum] -> Equal5/1
  Constant8/1 -> Equal4/2
  AND/1 -> OR/2
  [VTQD_RegenMode_enum] -> Equal4/1
  Equal5/1 -> AND/2
  Delay/1 -> OR/1
  OR/1 -> SR_Latch3/2
  Delay2/1 -> Equal6/1
  Constant12/1 -> Relational Operator/2
  [VTQD_OPDHoldR2D_flg] -> Delay3/1
  Constant13/1 -> Relational Operator1/2
  DelayEnable/1 -> SR_Latch4/2  "VTQD_R2DEnOPDHold_flg"
  [VVMC_EstSlope_Deg] -> Relational Operator1/1
  [task_time_s] -> DelayEnable/3
  [VTQD_GearActualPosn_enum] -> Delay2/1
  Constant11/1 -> Equal9/2
  [VTQD_GearActualPosn_enum] -> Equal9/1
  Constant14/1 -> Relational Operator2/2
  [VTQD_VehActSpd_kph] -> Relational Operator2/1
  AND4/1 -> DelayEnable/1
  Constant10/1 -> Equal6/2
  Relational Operator1/1 -> AND1/4
  AND1/1 -> SR_Latch4/1
  Relational Operator/1 -> AND1/3
  Constant15/1 -> DelayEnable/2
  Delay3/1 -> AND4/1
  [VVMC_EstSlope_Deg] -> Relational Operator/1
  Equal6/1 -> AND1/1
  SR_Latch4/1 -> [VTQD_OPDHoldR2D_flg]  "VTQD_OPDHoldR2D_flg"
  Equal9/1 -> AND1/2
  Relational Operator2/1 -> AND4/2
  [VTQD_VehActSpd_kph] -> Relational Operator3/1
  Relational Operator3/1 -> AND2/5
  OR1/1 -> AND2/3
  Constant6/1 -> Relational Operator3/2
  Equal3/1 -> AND2/6
  NOT3/1 -> AND2/1
  NOT4/1 -> AND2/4
  [VINP_ABSActive_flg] -> NOT6/1
  NOT6/1 -> AND2/10
  [VINP_ESCActive_flg] -> NOT5/1
  [VINP_EPBSta_enum] -> Equal3/1
  Constant7/1 -> Equal3/2
  NOT5/1 -> AND2/9
  [VINP_RrPTCSActive_flg] -> NOT2/1
  [VVMC_CruzActive_flg] -> NOT4/1
  AND3/1 -> OR1/1
  Equal2/1 -> AND3/1
  [VTQD_GearActualPosn_enum] -> Equal2/1
  NOT/1 -> AND3/2
  [VTQD_OPDHoldR2D_flg] -> NOT/1
  Constant5/1 -> Equal2/2
  [VTQD_AntiBlockEnOPDHold_flg] -> AND2/2
  [VTQD_OPDHoldDelayForP_flg] -> OR1/2
  [VVMC_ADASActive_flg] -> NOT3/1
  [VINP_FrPTCSActive_flg] -> NOT1/1
  VVMC_EstSlope_Deg/1 -> [VVMC_EstSlope_Deg]
  task_time_s/1 -> [task_time_s]
  VINP_ABSActive_flg/1 -> [VINP_ABSActive_flg]
  VINP_FrPTCSActive_flg/1 -> [VINP_FrPTCSActive_flg]
  VINP_ESCActive_flg/1 -> [VINP_ESCActive_flg]
  VINP_RrPTCSActive_flg/1 -> [VINP_RrPTCSActive_flg]
  NOT7/1 -> AND2/11
  [VVMC_APSActive_flg] -> NOT7/1
  VVMC_APSActive_flg/1 -> [VVMC_APSActive_flg]
  NOT8/1 -> AND7/2
  [VINP_IVICreepOnSW_flg] -> NOT8/1
  Constant40/1 -> Equal8/2
  [VTQD_OPDHoldRgnOn2Off_flg] -> OR5/1
  [VTQD_RegenMode_enum] -> Equal8/1
  AND7/1 -> OR5/3
  OR5/1 -> [VTQD_AntiBlockEnOPDHold_flg]  "VTQD_AntiBlockEnOPDHold_flg"
  Equal8/1 -> OR5/2
  [VTQD_PedAccTqEn_flg] -> AND7/1
  VINP_IVICreepOnSW_flg/1 -> [VINP_IVICreepOnSW_flg]
  VTQD_PedAccTqEn_flg/1 -> [VTQD_PedAccTqEn_flg]
  VTQD_IVIRockModeEn_flg/1 -> [VTQD_IVIRockModeEn_flg]
  [VTQD_IVIRockModeEn_flg] -> NOT9/1
  NOT9/1 -> AND2/12
  NOT2/1 -> AND2/8
  NOT1/1 -> AND2/7
  VTQD_SkipDirect_enum/1 -> [VTQD_SkipDirect_enum]
  VTQD_ActWhlSkipSta_enum/1 -> [VTQD_ActWhlSkipSta_enum]
  [VTQD_ActWhlSkipSta_enum] -> MTQD_WhlSkipDisOPDHold_Y_enum/1
  MTQD_WhlSkipDisOPDHold_Y_enum/1 -> [VTQD_WhlSkipDisOPDHold_enum]  "VTQD_WhlSkipDisOPDHold_enum"
  [VTQD_WhlSkipDisOPDHold_enum] -> Equal/1
  Constant16/1 -> Equal/2
  Constant17/1 -> Equal7/2
  [VTQD_SkipDirect_enum] -> Equal7/1
  Equal/1 -> AND8/1
  Equal7/1 -> AND8/2
  AND8/1 -> SR_Latch/1
  Constant19/1 -> Equal13/2
  [VTQD_WhlSkipDisOPDHold_enum] -> Equal13/1
  [VTQD_GearActualPosn_enum] -> Equal14/1
  [VTQD_GearActualPosn_enum] -> Equal15/1
  Constant21/1 -> Equal15/2
  Constant20/1 -> Equal14/2
  Equal14/1 -> OR3/1
  Equal15/1 -> OR3/2
  [task_time_s] -> DelayEnable1/3
  Constant22/1 -> DelayEnable1/2
  Relational Operator4/1 -> AND8/3
  [VTQD_VehActSpd_kph] -> Relational Operator4/1
  Constant18/1 -> Relational Operator4/2
  Constant23/1 -> Relational Operator5/2
  [VTQD_VehActSpd_kph] -> Relational Operator5/1
  Relational Operator5/1 -> OR3/3
  OR3/1 -> AND9/1
  Equal13/1 -> AND9/2
  AND9/1 -> DelayEnable1/1
  DelayEnable1/1 -> [VTQD_SkipDisOPDHoldReset_flg]  "VTQD_SkipDisOPDHoldReset_flg"
  [VTQD_SkipDisOPDHoldReset_flg] -> SR_Latch/2
  SR_Latch/1 -> [VTQD_WhlSkipDisOPDHold_flg]  "VTQD_WhlSkipDisOPDHold_flg"
  [VTQD_WhlSkipDisOPDHold_flg] -> NOT10/1
  NOT10/1 -> AND2/13
  [VTQD_LimpHomeAct_flg] -> NOT11/1
  NOT11/1 -> AND2/14
  VTQD_LimpHomeAct_flg/1 -> [VTQD_LimpHomeAct_flg]

== system tqd/TQD/TorqueDemand/TorqueModule/TqCoordination/Coordinate_ADAS ==
  VVMC_ADASWhlTqReq_Nm : Inport
  VTQD_PreLoadHold_flg : Inport  Port=2
  VTQD_DriverWhlTqDem_Nm : Inport  Port=3
  Action Port : ActionPort  ActionPortLabel=elseif( u3 ~= 0)
  Constant9 : Constant  Value=ENUM_TQSOURCE_ADAS
  Switch : Switch  Criteria=u2 > Threshold
  VTQD_ADASWhlTqReq_Nm : Outport
  VTQD_TqSourceADAS_enum : Outport  Port=2
  wires:
  VTQD_DriverWhlTqDem_Nm/1 -> Switch/1
  Switch/1 -> VTQD_ADASWhlTqReq_Nm/1
  VTQD_PreLoadHold_flg/1 -> Switch/2
  Constant9/1 -> VTQD_TqSourceADAS_enum/1
  VVMC_ADASWhlTqReq_Nm/1 -> Switch/3

== system tqd/TQD/TorqueDemand/TorqueModule/TqCoordination/Coordinate_ADASForceIdle ==
  Action Port : ActionPort  ActionPortLabel=elseif(u2 ~= 0)
  Constant : Constant  Value=ZERO_FLOAT
  Constant8 : Constant  Value=ENUM_TQSOURCE_ADASFORCEIDLE
  VTQD_ADASForceIdleReq_Nm : Outport
  VTQD_ADASForceIdle_enum : Outport  Port=2
  wires:
  Constant8/1 -> VTQD_ADASForceIdle_enum/1
  Constant/1 -> VTQD_ADASForceIdleReq_Nm/1

== system tqd/TQD/TorqueDemand/TorqueModule/TqCoordination/Coordinate_APS ==
  VTQD_DriverWhlTqDem_Nm : Inport
  Action Port : ActionPort  ActionPortLabel=elseif( u6 ~= 0)
  Constant9 : Constant  Value=ENUM_TQSOURCE_APS
  VTQD_APSWhlTqReq_Nm : Outport
  VTQD_TqSourceAPS_enum : Outport  Port=2
  wires:
  Constant9/1 -> VTQD_TqSourceAPS_enum/1
  VTQD_DriverWhlTqDem_Nm/1 -> VTQD_APSWhlTqReq_Nm/1

== system tqd/TQD/TorqueDemand/TorqueModule/TqCoordination/Coordinate_Cruise ==
  VVMC_CruzWhlTqReq_Nm : Inport
  Action Port : ActionPort  ActionPortLabel=elseif( u4 ~= 0)
  Constant9 : Constant  Value=ENUM_TQSOURCE_CC
  VTQD_CruzWhlTqReq_Nm : Outport
  VTQD_TqSourceCruz_enum : Outport  Port=2
  wires:
  Constant9/1 -> VTQD_TqSourceCruz_enum/1
  VVMC_CruzWhlTqReq_Nm/1 -> VTQD_CruzWhlTqReq_Nm/1

== system tqd/TQD/TorqueDemand/TorqueModule/TqCoordination/Coordinate_DirverPedal ==
  VTQD_DriverWhlTqDem_Nm : Inport
  Action Port : ActionPort  ActionPortLabel=else
  Constant9 : Constant  Value=ENUM_TQSOURCE_INTERNAL
  VTQD_DriverWhlTqReq_Nm : Outport
  VTQD_TqSourceInternal_enum : Outport  Port=2
  wires:
  VTQD_DriverWhlTqDem_Nm/1 -> VTQD_DriverWhlTqReq_Nm/1
  Constant9/1 -> VTQD_TqSourceInternal_enum/1

== system tqd/TQD/TorqueDemand/TorqueModule/TqCoordination/Coordinate_MSA ==
  VVMC_MSAWhlTqReq_Nm : Inport
  Action Port : ActionPort  ActionPortLabel=elseif( u5 ~= 0)
  Constant9 : Constant  Value=ENUM_TQSOURCE_MSA
  VTQD_MSAWhlTqReq_Nm : Outport
  VTQD_TqSourceMSA_enum : Outport  Port=2
  wires:
  Constant9/1 -> VTQD_TqSourceMSA_enum/1
  VVMC_MSAWhlTqReq_Nm/1 -> VTQD_MSAWhlTqReq_Nm/1

== system tqd/TQD/TorqueDemand/TorqueModule/TqCoordination/Coordinate_NoSuitbleGear_flg ==
  Action Port : ActionPort
  Constant5 : Constant  Value=KTQD_DriverTqDemN_Nm
  Constant8 : Constant  Value=ENUM_TQSOURCE_INVALID
  VTQD_GearNoSuitReq_Nm : Outport
  VTQD_TqSourceGearNoSuit_enum : Outport  Port=2
  wires:
  Constant5/1 -> VTQD_GearNoSuitReq_Nm/1
  Constant8/1 -> VTQD_TqSourceGearNoSuit_enum/1

== system tqd/TQD/TorqueDemand/TorqueModule/TqCoordination/Total Demand Capacity Torque  ==
  note: Total Comman Capacity Torque
  note: HV Available Output Torque Power
  VINP_HVBPwrAvailDchrg_kW : Inport
  VINP_HVBPwrAvailChrg_kW : Inport  Port=2
  VTQD_MotorLossTotal_kw : Inport  Port=3
  VTQD_FrShaftSpd_rpm : Inport  Port=4
  VTQD_RrShaftSpd_rpm : Inport  Port=5
  Abs{,1..6} (7 alike) : Abs
  Add : Sum
  Constant : Constant  Value=KTQD_DCDCCalPwrAvailRsv_kW
  Constant1 : Constant  Value=KTQD_THCMCalPwrAvailRsv_kW
  Constant2 : Constant  Value=KTQD_TMPwrAvailDchrg_kW_ovrdflg
  Constant3 : Constant  Value=ZERO_FLOAT
  Constant4 : Constant  Value=KTQD_BatapCont_factor
  Constant5 : Constant  Value=ONE_FLOAT
  Constant6 : Constant  Value=KTQD_BatapCont_factor
  Constant7 : Constant  Value=ONE_FLOAT
  Delay : Delay  DelayLength=1  InitialCondition=single(0)
      settings: AttributesFormatString=%<InitialCondition>
  Fcn : Fcn  Expr=u[1]/u[2]/pi*u[3]
  Fcn1 : Fcn  Expr=u[1]/u[2]/pi*u[3]
  Gain4 : Gain  Gain=MINUSONE_FLOAT
  Max : MinMax  Function=max  Inputs=2
  Max1 : MinMax  Function=max  Inputs=3
  Max2 : MinMax  Function=max  Inputs=3
  Mux : Mux  Inputs=3
  Mux1 : Mux  Inputs=3
  Saturation1 : Saturate  UpperLimit=ZERO_FLOAT  LowerLimit=KTQD_TotalLowTheldTrq_Nm
      settings: AttributesFormatString=|
      | Upper Limit :%<UpperLimit>
      | Lower Limit :%<LowerLimit>
  Saturation2 : Saturate  UpperLimit=KTQD_TotalUpTheldTrq_Nm  LowerLimit=ZERO_FLOAT
      settings: AttributesFormatString=|
      | Upper Limit :%<UpperLimit>
      | Lower Limit :%<LowerLimit>
  Subtract : Sum  Inputs=+--
  Switch : Switch  Criteria=u2 ~= 0
      settings: AttributesFormatString=%<Criteria>
  VTQD_TotalWhlTqCapMot_Nm : Outport
  VTQD_TotalWhlTqCapGen_Nm : Outport  Port=2
  wires:
  Constant1/1 -> Add/2
  Constant/1 -> Add/1
  Add/1 -> Subtract/2
  Subtract/1 -> Max/1
  Constant3/1 -> Max/2
  Max/1 -> Switch/1
  Constant2/1 -> Switch/2
  [VINP_HVBPwrAvailDchrg_kW] -> Abs1/1
  Switch/1 -> [VTQD_TotalAvailDchrg_kW]  "VTQD_TotalAvailDchrg_kW"
  [VINP_HVBPwrAvailDchrg_kW] -> Abs/1
  Abs/1 -> Subtract/1
  Abs1/1 -> Switch/3
  [VTQD_FrShaftSpd_rpm] -> Abs2/1
  [VTQD_RrShaftSpd_rpm] -> Abs3/1
  Abs2/1 -> Max1/1
  Abs3/1 -> Max1/2
  Max1/1 -> Mux/2
  [VTQD_TotalAvailDchrg_kW] -> Mux/1
  Constant4/1 -> Mux/3
  Mux/1 -> Fcn/1
  Fcn/1 -> Saturation2/1
  Constant5/1 -> Max1/3
  Max2/1 -> Mux1/2
  Abs5/1 -> Max2/2
  Mux1/1 -> Fcn1/1
  Constant6/1 -> Mux1/3
  Abs4/1 -> Max2/1
  [VTQD_RrShaftSpd_rpm] -> Abs5/1
  Constant7/1 -> Max2/3
  [VTQD_FrShaftSpd_rpm] -> Abs4/1
  Abs6/1 -> Mux1/1
  [VINP_HVBPwrAvailChrg_kW] -> Abs6/1
  Gain4/1 -> Saturation1/1
  Fcn1/1 -> Gain4/1
  Saturation1/1 -> [VTQD_TotalWhlTqCapGen_Nm]  "VTQD_TotalWhlTqCapGen_Nm"
  Saturation2/1 -> [VTQD_TotalWhlTqCapMot_Nm]  "VTQD_TotalWhlTqCapMot_Nm"
  VINP_HVBPwrAvailDchrg_kW/1 -> [VINP_HVBPwrAvailDchrg_kW]
  VINP_HVBPwrAvailChrg_kW/1 -> [VINP_HVBPwrAvailChrg_kW]
  VTQD_MotorLossTotal_kw/1 -> [VTQD_MotorLossTotal_kw]
  VTQD_FrShaftSpd_rpm/1 -> [VTQD_FrShaftSpd_rpm]
  VTQD_RrShaftSpd_rpm/1 -> [VTQD_RrShaftSpd_rpm]
  [VTQD_TotalWhlTqCapMot_Nm] -> VTQD_TotalWhlTqCapMot_Nm/1
  [VTQD_TotalWhlTqCapGen_Nm] -> VTQD_TotalWhlTqCapGen_Nm/1
  Delay/1 -> Subtract/3
  [VTQD_MotorLossTotal_kw] -> Delay/1

== system tqd/TQD/TorqueDemand/TorqueModule/TqDistribution/AWD_Ratio ==
  VVMC_APSActive_flg : Inport
  VTQD_CreepPrLoadEnable_flg : Inport  Port=2
  VTQD_RrRatioWithRrSR_rat : Inport  Port=3
  VTQD_CreepEnable_flg : Inport  Port=4
  VTQD_OrigRrDriverRatio_rat : Inport  Port=5
  VTQD_CreepRrTqSpRat_rat : Inport  Port=6
  VTQD_RrTqSRRateTs_c : Inport  Port=7
  task_time_s : Inport  Port=8
  Action Port : ActionPort
  AND : Logic  AllPortsSameDT=off  OutDataTypeStr=boolean
  AND2 : Logic  AllPortsSameDT=off  OutDataTypeStr=boolean
  Constant : Constant  Value=ONE_FLOAT
  Constant10 : Constant  Value=KTQD_AWDRrRatio_rat_ovrdflg  VectorParams1D=off  SampleTime=-1
  Constant11 : Constant  Value=KTQD_AWDRrRatio_rat_ovrdval  VectorParams1D=off  SampleTime=-1
  Constant12 : Constant  Value=KTQD_DrvSelPwrTrainSW_flg  VectorParams1D=off  SampleTime=-1
  Constant14 : Constant  Value=KTQD_CreepWhlRatioSW_flg
  Constant17 : Constant  Value=KTQD_AWDTqRatioSW_enum
  Constant18 : Constant  Value=KTQD_DriverSelPowerTrain_enum
  Constant19 : Constant  OutDataTypeStr=uint8
  Constant20 : Constant  Value=KTQD_AWDTqRatioSW_enum
  Constant21 : Constant  Value=2  OutDataTypeStr=uint8
  Constant3 : Constant  Value=ENUM_DRIVETRAIN_FWD  VectorParams1D=off  SampleTime=-1
  Constant4 : Constant  Value=ENUM_DRIVETRAIN_AWD  VectorParams1D=off  SampleTime=-1
  Constant6 : Constant  Value=KTQD_AWDFWDSelRRatio_rat  VectorParams1D=off  SampleTime=-1
  Constant7 : Constant  Value=KTQD_AWDRWDSelRRatio_rat  VectorParams1D=off  SampleTime=-1
  Constant8 : Constant  Value=KTQD_AWDFrRatio_rat_ovrdflg  VectorParams1D=off  SampleTime=-1
  Constant9 : Constant  Value=KTQD_AWDFrRatio_rat_ovrdval  VectorParams1D=off  SampleTime=-1
  Equal1 : RelationalOperator  Operator=~=  OutDataTypeStr=boolean  RndMeth=Simplest
  Equal3 : RelationalOperator  Operator===  OutDataTypeStr=boolean  RndMeth=Simplest
  Equal6 : RelationalOperator  Operator===  OutDataTypeStr=boolean  RndMeth=Simplest
  Equal7 : RelationalOperator  Operator===  OutDataTypeStr=boolean  RndMeth=Simplest
  FirstOrderFilter : hcu_lib/Basic_Blocks/FirstOrderFilter
  LiuzgSwitch2 : Switch  Criteria=u2 ~= 0
      settings: AttributesFormatString=<%<Criteria>>
  LiuzgSwitch4 : Switch  Criteria=u2 ~= 0
      settings: AttributesFormatString=<%<Criteria>>
  LiuzgSwitch5 : Switch  Criteria=u2 ~= 0
      settings: AttributesFormatString=<%<Criteria>>
  OR : Logic  Operator=OR  AllPortsSameDT=off  OutDataTypeStr=boolean
  OR1 : Logic  AllPortsSameDT=off  OutDataTypeStr=boolean
  OR3 : Logic  Operator=OR  AllPortsSameDT=off  OutDataTypeStr=boolean
  Saturation : Saturate  UpperLimit=KTQD_RrEDUTqDistrictMax_gain  LowerLimit=KTQD_RrEDUTqDistrictMin_gain
      settings: AttributesFormatString=|
      | <%<UpperLimit>>
      | <%<LowerLimit>>
  Subtract : Sum  Inputs=+-
  Switch : Switch  Criteria=u2 > Threshold
  Switch1 : Switch  Criteria=u2 > Threshold
  Switch3 : Switch  Criteria=u2 > Threshold
  VTQD_FrRatio_AWD : Outport
  VTQD_RrRatio_AWD : Outport  Port=2
  wires:
  Constant/1 -> Subtract/1
  Saturation/1 -> Switch1/3, Subtract/2
  OR/1 -> OR1/1
  [VTQD_CreepPrLoadEnable_flg] -> OR/2
  [VVMC_APSActive_flg] -> OR/1
  VVMC_APSActive_flg/1 -> [VVMC_APSActive_flg]
  VTQD_CreepPrLoadEnable_flg/1 -> [VTQD_CreepPrLoadEnable_flg]
  [VINP_DriverSelPowerTrain_enum] -> Equal1/1
  Constant4/1 -> Equal1/2
  LiuzgSwitch5/1 -> LiuzgSwitch4/1
  Constant3/1 -> Equal3/2
  [VINP_DriverSelPowerTrain_enum] -> Equal3/1
  Equal3/1 -> LiuzgSwitch5/2
  LiuzgSwitch4/1 -> Saturation/1
  Constant18/1 -> [VINP_DriverSelPowerTrain_enum]  "VINP_DriverSelPowerTrain_enum"
  Subtract/1 -> Switch/3
  Switch/1 -> VTQD_FrRatio_AWD/1
  Switch1/1 -> VTQD_RrRatio_AWD/1
  Constant8/1 -> Switch/2
  Constant9/1 -> Switch/1
  Constant11/1 -> Switch1/1
  Constant10/1 -> Switch1/2
  Constant12/1 -> AND/2
  Equal1/1 -> AND/1
  AND/1 -> LiuzgSwitch4/2
  OR1/1 -> LiuzgSwitch2/2
  Constant14/1 -> OR1/2
  VTQD_CreepEnable_flg/1 -> [VTQD_CreepEnable_flg]
  VTQD_RrRatioWithRrSR_rat/1 -> [VTQD_RrRatioWithRrSR_rat]
  Constant7/1 -> LiuzgSwitch5/3
  Constant6/1 -> LiuzgSwitch5/1
  Switch3/1 -> LiuzgSwitch2/3  "VTQD_FitRrDriverRatio_rat"
  [VTQD_OrigRrDriverRatio_rat] -> Switch3/3
  [VTQD_RrRatioWithRrSR_rat] -> Switch3/1
  Constant17/1 -> Equal6/1
  Constant19/1 -> Equal6/2
  Equal6/1 -> AND2/1
  [VTQD_CreepEnable_flg] -> AND2/2
  AND2/1 -> OR3/1
  Constant21/1 -> Equal7/2
  Constant20/1 -> Equal7/1
  Equal7/1 -> OR3/2
  OR3/1 -> Switch3/2
  VTQD_OrigRrDriverRatio_rat/1 -> [VTQD_OrigRrDriverRatio_rat]
  VTQD_CreepRrTqSpRat_rat/1 -> [VTQD_CreepRrTqSpRat_rat]
  [VTQD_CreepRrTqSpRat_rat] -> LiuzgSwitch2/1
  VTQD_RrTqSRRateTs_c/1 -> [VTQD_RrTqSRRateTs_c]
  task_time_s/1 -> [task_time_s]
  LiuzgSwitch2/1 -> FirstOrderFilter/1
  FirstOrderFilter/1 -> LiuzgSwitch4/3
  [task_time_s] -> FirstOrderFilter/2
  [VTQD_RrTqSRRateTs_c] -> FirstOrderFilter/3

== system tqd/TQD/TorqueDemand/TorqueModule/TqDistribution/FWD_Ratio ==
  Action Port : ActionPort
  Constant : Constant  Value=ONE_FLOAT
  Constant1 : Constant  Value=ZERO_FLOAT
  VTQD_FrRatio_FWD : Outport
  VTQD_RrRatio_FWD : Outport  Port=2
  wires:
  Constant/1 -> VTQD_FrRatio_FWD/1
  Constant1/1 -> VTQD_RrRatio_FWD/1
